simulink model "gm_final_heart_sym2_level3_hdl"  (R2021a)
settings: Solver=FixedStepDiscrete  StartTime=0.0  StopTime=10.0  RelTol=1e-3
libraries: hdlmdlgenlib x34
(part 1 of 3)
settings Model: Creator=Acer  LastModifiedBy=Acer
settings OptimizationCC: BlockReduction=off  ConditionallyExecuteInputs=off  DefaultParameterBehavior=Inlined
settings DebuggingCC: AlgebraicLoopMsg=error  InheritedTsInSrcMsg=none  SingleTaskRateTransMsg=error
settings HardwareCC: ProdBitPerPointer=32  ProdBitPerSizeT=32  ProdBitPerPtrDiffT=32  ProdLargestAtomicFloat=None  ProdIntDivRoundTo=Undefined  ProdEndianess=Unspecified  ProdWordSize=32  ProdHWDeviceType=ASIC/FPGA->ASIC/FPGA  TargetBitPerPointer=64  TargetBitPerSizeT=64  TargetBitPerPtrDiffT=64  TargetLongLongMode=on  TargetIntDivRoundTo=Zero  TargetEndianess=LittleEndian  TargetWordSize=64  TargetHWDeviceType=Custom Processor->MATLAB Host Computer  ProdEqTarget=off

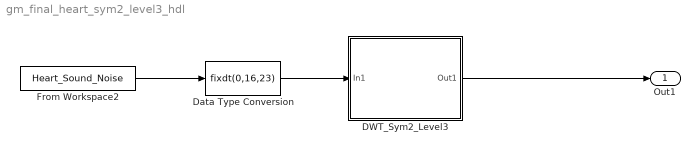
== system gm_final_heart_sym2_level3_hdl ==
  DWT_Sym2_Level3 : Subsystem
  Data Type Conversion : DataTypeConversion  OutDataTypeStr=fixdt(0,16,23)
  From Workspace2 : FromWorkspace  VariableName=Heart_Sound_Noise  OutDataTypeStr=double  SampleTime=1/44100
  Out1 : Outport  OutDataTypeStr=fixdt(1,16,22)
  wires:
  Data Type Conversion/1 -> DWT_Sym2_Level3/1(In1)
  DWT_Sym2_Level3/1(Out1) -> Out1/1
  From Workspace2/1 -> Data Type Conversion/1

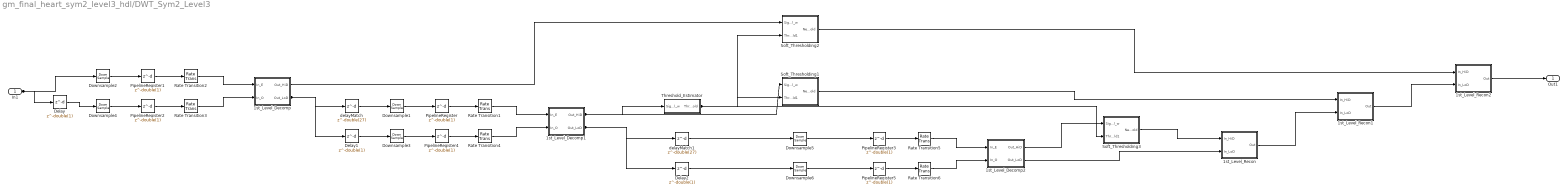
== system gm_final_heart_sym2_level3_hdl/DWT_Sym2_Level3 ==
  In1 : Inport  OutDataTypeStr=fixdt(0, 16, 23)  PortDimensions=1  SampleTime=2.26757369614512e-05
  1st_Level_Decomp : Subsystem
  1st_Level_Decomp1 : Subsystem
  1st_Level_Decomp2 : Subsystem
  1st_Level_Recon : Subsystem
  1st_Level_Recon1 : Subsystem
  1st_Level_Recon2 : Subsystem
  Delay : Delay  DelayLength=double(1)  InitialCondition=0  SampleTime=2.26757369614512e-05
  Delay1 : Delay  DelayLength=double(1)  InitialCondition=0  SampleTime=2.26757369614512e-05
  Delay2 : Delay  DelayLength=double(1)  InitialCondition=0  SampleTime=2.26757369614512e-05
  Downsample{1..2,4..5} (4 alike) : DownSample  N=double(30)  phase=double(0)  RateOptions=Allow multirate processing
  Downsample3 : DownSample  N=double(30)  phase=double(3)  RateOptions=Allow multirate processing
  Downsample6 : DownSample  N=double(30)  phase=double(3)  RateOptions=Allow multirate processing
  PipelineRegister{,1..5} (6 alike) : Delay  DelayLength=double(1)  InitialCondition=0  SampleTime=0.000680272108843537
  Rate Transition{1..6} (6 alike) : RateTransition  InitialCondition=double(0)  OutPortSampleTimeOpt=Multiple of input port sample time  OutPortSampleTimeMultiple=1/30
  Soft_Thresholding1 : Subsystem
  Soft_Thresholding2 : Subsystem
  Soft_Thresholding3 : Subsystem
  Threshold_Estimator : Subsystem
  delayMatch : Delay  DelayLength=double(27)  InitialCondition=0  SampleTime=2.26757369614512e-05
  delayMatch1 : Delay  DelayLength=double(27)  InitialCondition=0  SampleTime=2.26757369614512e-05
  Out1 : Outport  OutDataTypeStr=fixdt(1,16,22)  SampleTime=2.26757369614512e-05
  wires:
  In1/1 -> Downsample2/1, Delay/1
  1st_Level_Decomp/1(Out_HiD) -> Soft_Thresholding2/1(Signal_w)
  delayMatch/1 -> Downsample1/1
  1st_Level_Decomp1/1(Out_HiD) -> Soft_Thresholding1/1(Signal_w), Threshold_Estimator/1(Signal_w)
  delayMatch1/1 -> Downsample5/1
  1st_Level_Decomp2/1(Out_HiD) -> Soft_Thresholding3/1(Signal_w)
  1st_Level_Decomp2/2(Out_LoD) -> 1st_Level_Recon/2(In_LoD)
  1st_Level_Recon/1(Out) -> 1st_Level_Recon1/2(In_LoD)
  1st_Level_Recon1/1(Out) -> 1st_Level_Recon2/2(In_LoD)
  1st_Level_Recon2/1(Out) -> Out1/1
  Delay/1 -> Downsample4/1
  PipelineRegister/1 -> Rate Transition1/1
  PipelineRegister1/1 -> Rate Transition2/1
  PipelineRegister4/1 -> Rate Transition4/1
  PipelineRegister2/1 -> Rate Transition3/1
  PipelineRegister3/1 -> Rate Transition5/1
  PipelineRegister5/1 -> Rate Transition6/1
  Rate Transition1/1 -> 1st_Level_Decomp1/1(In_E)
  Rate Transition2/1 -> 1st_Level_Decomp/1(In_E)
  Rate Transition3/1 -> 1st_Level_Decomp/2(In_O)
  Rate Transition4/1 -> 1st_Level_Decomp1/2(In_O)
  Rate Transition5/1 -> 1st_Level_Decomp2/1(In_E)
  Rate Transition6/1 -> 1st_Level_Decomp2/2(In_O)
  Soft_Thresholding1/1(New_Threshold) -> 1st_Level_Recon1/1(In_HiD)
  Soft_Thresholding2/1(New_Threshold) -> 1st_Level_Recon2/1(In_HiD)
  Soft_Thresholding3/1(New_Threshold) -> 1st_Level_Recon/1(In_HiD)
  Threshold_Estimator/1(Threshold) -> Soft_Thresholding3/2(Threshold1), Soft_Thresholding2/2(Threshold1), Soft_Thresholding1/2(Threshold1)
  1st_Level_Decomp/2(Out_LoD) -> delayMatch/1, Delay1/1
  Delay1/1 -> Downsample3/1
  1st_Level_Decomp1/2(Out_LoD) -> delayMatch1/1, Delay2/1
  Delay2/1 -> Downsample6/1
  Downsample1/1 -> PipelineRegister/1
  Downsample2/1 -> PipelineRegister1/1
  Downsample4/1 -> PipelineRegister2/1
  Downsample5/1 -> PipelineRegister3/1
  Downsample3/1 -> PipelineRegister4/1
  Downsample6/1 -> PipelineRegister5/1

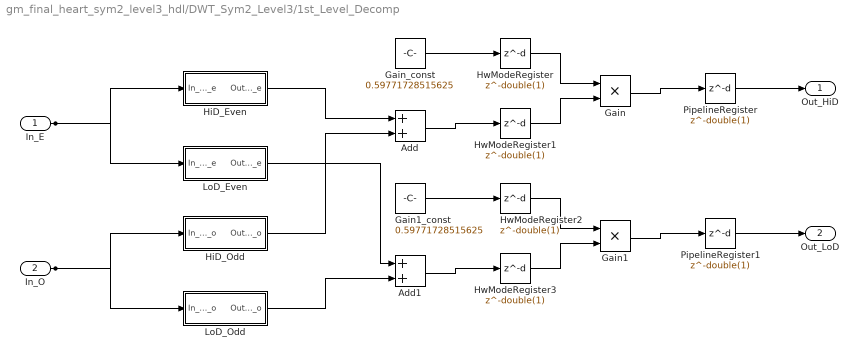
== system gm_final_heart_sym2_level3_hdl/DWT_Sym2_Level3/1st_Level_Decomp ==
  In_E : Inport  OutDataTypeStr=fixdt(0, 16, 23)  PortDimensions=1  SampleTime=2.26757369614512e-05
  In_O : Inport  Port=2  OutDataTypeStr=fixdt(0, 16, 23)  PortDimensions=1  SampleTime=2.26757369614512e-05
  Add : Sum  AccumDataTypeStr=fixdt(1, 16, 23)  OutDataTypeStr=fixdt(1, 16, 24)  SampleTime=2.26757369614512e-05
  Add1 : Sum  AccumDataTypeStr=fixdt(1, 16, 22)  OutDataTypeStr=fixdt(1, 16, 22)  SampleTime=2.26757369614512e-05
  Gain : Product  Inputs=**  OutDataTypeStr=fixdt(1, 16, 24)  SampleTime=2.26757369614512e-05
  Gain1 : Product  Inputs=**  OutDataTypeStr=fixdt(1, 16, 22)  SampleTime=2.26757369614512e-05
  Gain1_const : Constant  Value=0.59771728515625  OutDataTypeStr=fixdt(0, 16, 16)  SampleTime=2.26757369614512e-05
  Gain_const : Constant  Value=0.59771728515625  OutDataTypeStr=fixdt(0, 16, 16)  SampleTime=2.26757369614512e-05
  HiD_Even : Subsystem
  HiD_Odd : Subsystem
  HwModeRegister{,1..3} (4 alike) : Delay  DelayLength=double(1)  InitialCondition=0  SampleTime=2.26757369614512e-05
  LoD_Even : Subsystem
  LoD_Odd : Subsystem
  PipelineRegister : Delay  DelayLength=double(1)  InitialCondition=0  SampleTime=2.26757369614512e-05
  PipelineRegister1 : Delay  DelayLength=double(1)  InitialCondition=0  SampleTime=2.26757369614512e-05
  Out_HiD : Outport  OutDataTypeStr=fixdt(1,16,24)  SampleTime=2.26757369614512e-05
  Out_LoD : Outport  Port=2  OutDataTypeStr=fixdt(1,16,22)  SampleTime=2.26757369614512e-05
  wires:
  Add/1 -> HwModeRegister1/1
  Add1/1 -> HwModeRegister3/1
  PipelineRegister/1 -> Out_HiD/1
  PipelineRegister1/1 -> Out_LoD/1
  HiD_Even/1(Out_HiD_e) -> Add/1
  HiD_Odd/1(Out_HiD_o) -> Add/2
  LoD_Even/1(Out_LoD_e) -> Add1/1
  LoD_Odd/1(Out_LoD_o) -> Add1/2
  Gain_const/1 -> HwModeRegister/1
  Gain1_const/1 -> HwModeRegister2/1
  In_E/1 -> HiD_Even/1(In_HiD_e), LoD_Even/1(In_LoD_e)
  In_O/1 -> HiD_Odd/1(In_HiD_o), LoD_Odd/1(In_LoD_o)
  Gain/1 -> PipelineRegister/1
  HwModeRegister/1 -> Gain/1
  HwModeRegister1/1 -> Gain/2
  Gain1/1 -> PipelineRegister1/1
  HwModeRegister2/1 -> Gain1/1
  HwModeRegister3/1 -> Gain1/2

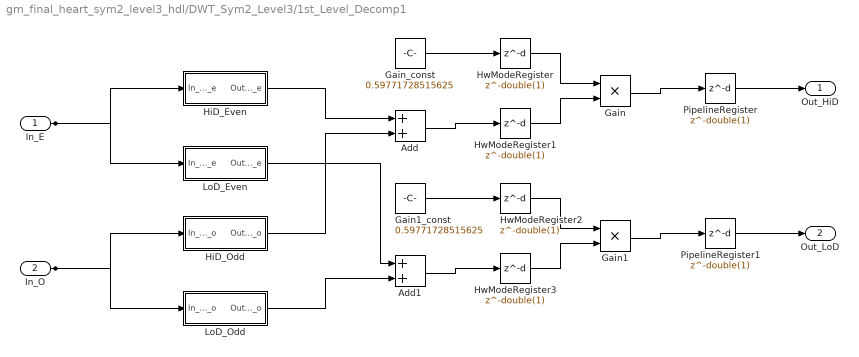
== system gm_final_heart_sym2_level3_hdl/DWT_Sym2_Level3/1st_Level_Decomp1 ==
  In_E : Inport  OutDataTypeStr=fixdt(1, 16, 22)  PortDimensions=1  SampleTime=2.26757369614512e-05
  In_O : Inport  Port=2  OutDataTypeStr=fixdt(1, 16, 22)  PortDimensions=1  SampleTime=2.26757369614512e-05
  Add : Sum  AccumDataTypeStr=fixdt(1, 16, 23)  OutDataTypeStr=fixdt(1, 16, 26)  SampleTime=2.26757369614512e-05
  Add1 : Sum  AccumDataTypeStr=fixdt(1, 16, 22)  OutDataTypeStr=fixdt(0, 16, 23)  SampleTime=2.26757369614512e-05
  Gain : Product  Inputs=**  OutDataTypeStr=fixdt(1, 16, 26)  SampleTime=2.26757369614512e-05
  Gain1 : Product  Inputs=**  OutDataTypeStr=fixdt(0, 16, 24)  SampleTime=2.26757369614512e-05
  Gain1_const : Constant  Value=0.59771728515625  OutDataTypeStr=fixdt(0, 16, 16)  SampleTime=2.26757369614512e-05
  Gain_const : Constant  Value=0.59771728515625  OutDataTypeStr=fixdt(0, 16, 16)  SampleTime=2.26757369614512e-05
  HiD_Even : Subsystem
  HiD_Odd : Subsystem
  HwModeRegister{,1..3} (4 alike) : Delay  DelayLength=double(1)  InitialCondition=0  SampleTime=2.26757369614512e-05
  LoD_Even : Subsystem
  LoD_Odd : Subsystem
  PipelineRegister : Delay  DelayLength=double(1)  InitialCondition=0  SampleTime=2.26757369614512e-05
  PipelineRegister1 : Delay  DelayLength=double(1)  InitialCondition=0  SampleTime=2.26757369614512e-05
  Out_HiD : Outport  OutDataTypeStr=fixdt(1,16,26)  SampleTime=2.26757369614512e-05
  Out_LoD : Outport  Port=2  OutDataTypeStr=fixdt(0,16,24)  SampleTime=2.26757369614512e-05
  wires:
  Add/1 -> HwModeRegister1/1
  Add1/1 -> HwModeRegister3/1
  PipelineRegister/1 -> Out_HiD/1
  PipelineRegister1/1 -> Out_LoD/1
  HiD_Even/1(Out_HiD_e) -> Add/1
  HiD_Odd/1(Out_HiD_o) -> Add/2
  LoD_Even/1(Out_LoD_e) -> Add1/1
  LoD_Odd/1(Out_LoD_o) -> Add1/2
  Gain_const/1 -> HwModeRegister/1
  Gain1_const/1 -> HwModeRegister2/1
  In_E/1 -> HiD_Even/1(In_HiD_e), LoD_Even/1(In_LoD_e)
  In_O/1 -> HiD_Odd/1(In_HiD_o), LoD_Odd/1(In_LoD_o)
  Gain/1 -> PipelineRegister/1
  HwModeRegister/1 -> Gain/1
  HwModeRegister1/1 -> Gain/2
  Gain1/1 -> PipelineRegister1/1
  HwModeRegister2/1 -> Gain1/1
  HwModeRegister3/1 -> Gain1/2

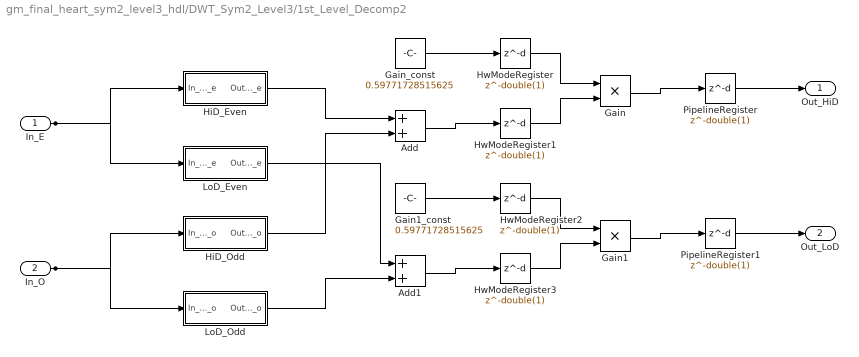
== system gm_final_heart_sym2_level3_hdl/DWT_Sym2_Level3/1st_Level_Decomp2 ==
  In_E : Inport  OutDataTypeStr=fixdt(0, 16, 24)  PortDimensions=1  SampleTime=2.26757369614512e-05
  In_O : Inport  Port=2  OutDataTypeStr=fixdt(0, 16, 24)  PortDimensions=1  SampleTime=2.26757369614512e-05
  Add : Sum  AccumDataTypeStr=fixdt(1, 16, 23)  OutDataTypeStr=fixdt(1, 16, 26)  SampleTime=2.26757369614512e-05
  Add1 : Sum  AccumDataTypeStr=fixdt(1, 16, 22)  OutDataTypeStr=fixdt(0, 16, 23)  SampleTime=2.26757369614512e-05
  Gain : Product  Inputs=**  OutDataTypeStr=fixdt(1, 16, 27)  SampleTime=2.26757369614512e-05
  Gain1 : Product  Inputs=**  OutDataTypeStr=fixdt(0, 16, 24)  SampleTime=2.26757369614512e-05
  Gain1_const : Constant  Value=0.59771728515625  OutDataTypeStr=fixdt(0, 16, 16)  SampleTime=2.26757369614512e-05
  Gain_const : Constant  Value=0.59771728515625  OutDataTypeStr=fixdt(0, 16, 16)  SampleTime=2.26757369614512e-05
  HiD_Even : Subsystem
  HiD_Odd : Subsystem
  HwModeRegister{,1..3} (4 alike) : Delay  DelayLength=double(1)  InitialCondition=0  SampleTime=2.26757369614512e-05
  LoD_Even : Subsystem
  LoD_Odd : Subsystem
  PipelineRegister : Delay  DelayLength=double(1)  InitialCondition=0  SampleTime=2.26757369614512e-05
  PipelineRegister1 : Delay  DelayLength=double(1)  InitialCondition=0  SampleTime=2.26757369614512e-05
  Out_HiD : Outport  OutDataTypeStr=fixdt(1,16,27)  SampleTime=2.26757369614512e-05
  Out_LoD : Outport  Port=2  OutDataTypeStr=fixdt(0,16,24)  SampleTime=2.26757369614512e-05
  wires:
  Add/1 -> HwModeRegister1/1
  Add1/1 -> HwModeRegister3/1
  PipelineRegister/1 -> Out_HiD/1
  PipelineRegister1/1 -> Out_LoD/1
  HiD_Even/1(Out_HiD_e) -> Add/1
  HiD_Odd/1(Out_HiD_o) -> Add/2
  LoD_Even/1(Out_LoD_e) -> Add1/1
  LoD_Odd/1(Out_LoD_o) -> Add1/2
  Gain_const/1 -> HwModeRegister/1
  Gain1_const/1 -> HwModeRegister2/1
  In_E/1 -> HiD_Even/1(In_HiD_e), LoD_Even/1(In_LoD_e)
  In_O/1 -> HiD_Odd/1(In_HiD_o), LoD_Odd/1(In_LoD_o)
  Gain/1 -> PipelineRegister/1
  HwModeRegister/1 -> Gain/1
  HwModeRegister1/1 -> Gain/2
  Gain1/1 -> PipelineRegister1/1
  HwModeRegister2/1 -> Gain1/1
  HwModeRegister3/1 -> Gain1/2

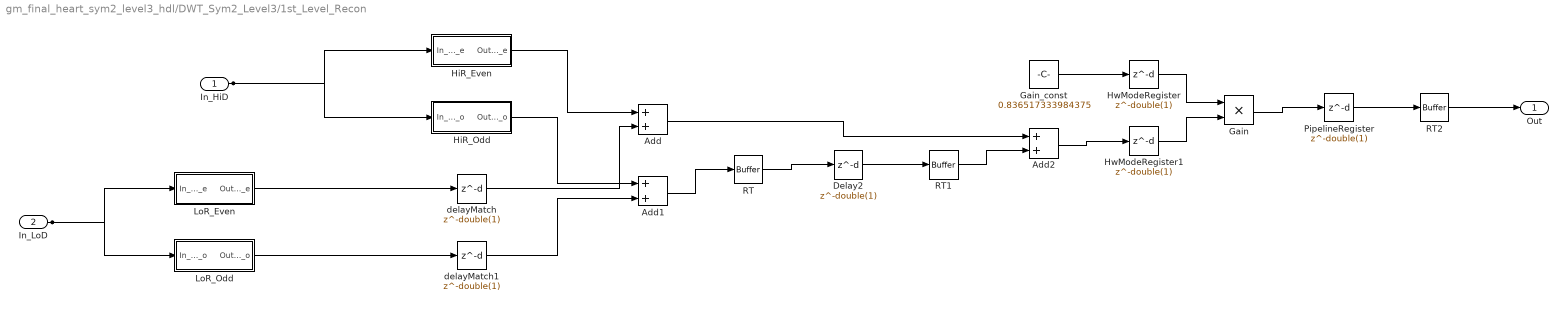
== system gm_final_heart_sym2_level3_hdl/DWT_Sym2_Level3/1st_Level_Recon ==
  In_HiD : Inport  OutDataTypeStr=fixdt(1, 16, 27)  PortDimensions=1  SampleTime=2.26757369614512e-05
  In_LoD : Inport  Port=2  OutDataTypeStr=fixdt(0, 16, 24)  PortDimensions=1  SampleTime=2.26757369614512e-05
  Add : Sum  AccumDataTypeStr=fixdt(1, 16, 23)  OutDataTypeStr=fixdt(1, 16, 23)  SampleTime=2.26757369614512e-05
  Add1 : Sum  AccumDataTypeStr=fixdt(1, 16, 23)  OutDataTypeStr=fixdt(1, 16, 23)  SampleTime=2.26757369614512e-05
  Add2 : Sum  AccumDataTypeStr=fixdt(1, 16, 22)  OutDataTypeStr=fixdt(1, 16, 22)  SampleTime=2.26757369614512e-05
  Delay2 : Delay  DelayLength=double(1)  InitialCondition=0  SampleTime=2.26757369614512e-05
  Gain : Product  Inputs=**  OutDataTypeStr=fixdt(1, 16, 23)  SampleTime=2.26757369614512e-05
  Gain_const : Constant  Value=0.836517333984375  OutDataTypeStr=fixdt(0, 16, 16)  SampleTime=2.26757369614512e-05
  HiR_Even : Subsystem
  HiR_Odd : Subsystem
  HwModeRegister : Delay  DelayLength=double(1)  InitialCondition=0  SampleTime=2.26757369614512e-05
  HwModeRegister1 : Delay  DelayLength=double(1)  InitialCondition=0  SampleTime=2.26757369614512e-05
  LoR_Even : Subsystem
  LoR_Odd : Subsystem
  PipelineRegister : Delay  DelayLength=double(1)  InitialCondition=0  SampleTime=2.26757369614512e-05
  RT : hdlmdlgenlib/Buffer
      settings: SourceProductBaseCode=SL
  RT1 : hdlmdlgenlib/Buffer
      settings: SourceProductBaseCode=SL
  RT2 : hdlmdlgenlib/Buffer
      settings: SourceProductBaseCode=SL
  delayMatch : Delay  DelayLength=double(1)  InitialCondition=0  SampleTime=2.26757369614512e-05
  delayMatch1 : Delay  DelayLength=double(1)  InitialCondition=0  SampleTime=2.26757369614512e-05
  Out : Outport  OutDataTypeStr=fixdt(1,16,23)  SampleTime=2.26757369614512e-05
  wires:
  Add/1 -> Add2/1
  Add1/1 -> RT/1
  Add2/1 -> HwModeRegister1/1
  Delay2/1 -> RT1/1
  PipelineRegister/1 -> RT2/1
  HiR_Even/1(Out_HiR_e) -> Add/1
  HiR_Odd/1(Out_HiR_o) -> Add1/1
  delayMatch/1 -> Add/2
  delayMatch1/1 -> Add1/2
  RT/1 -> Delay2/1
  RT1/1 -> Add2/2
  RT2/1 -> Out/1
  Gain_const/1 -> HwModeRegister/1
  In_HiD/1 -> HiR_Even/1(In_HiR_e), HiR_Odd/1(In_HiR_o)
  In_LoD/1 -> LoR_Odd/1(In_LoR_o), LoR_Even/1(In_LoR_e)
  LoR_Even/1(Out_LoR_e) -> delayMatch/1
  LoR_Odd/1(Out_HiR_o) -> delayMatch1/1
  Gain/1 -> PipelineRegister/1
  HwModeRegister/1 -> Gain/1
  HwModeRegister1/1 -> Gain/2

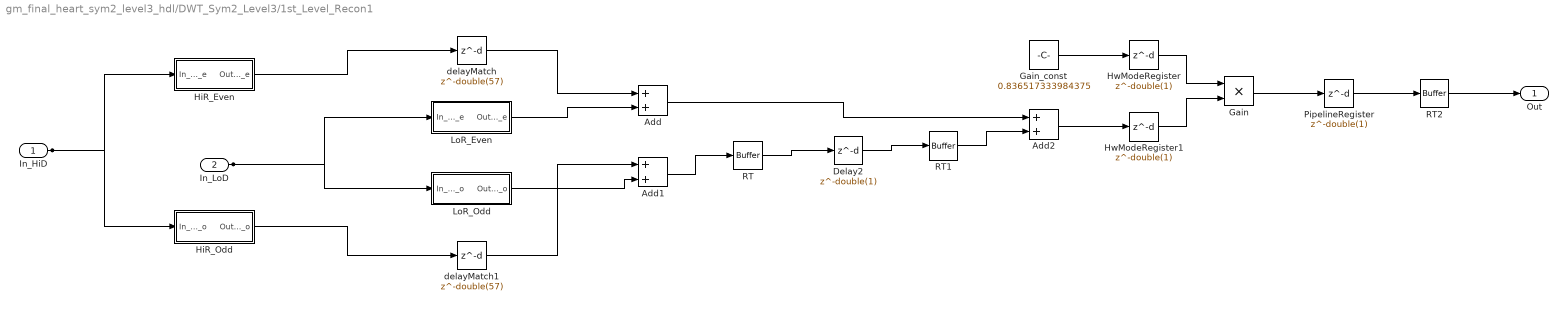
== system gm_final_heart_sym2_level3_hdl/DWT_Sym2_Level3/1st_Level_Recon1 ==
  In_HiD : Inport  OutDataTypeStr=fixdt(1, 16, 27)  PortDimensions=1  SampleTime=2.26757369614512e-05
  In_LoD : Inport  Port=2  OutDataTypeStr=fixdt(1, 16, 23)  PortDimensions=1  SampleTime=2.26757369614512e-05
  Add : Sum  AccumDataTypeStr=fixdt(1, 16, 23)  OutDataTypeStr=fixdt(1, 16, 23)  SampleTime=2.26757369614512e-05
  Add1 : Sum  AccumDataTypeStr=fixdt(1, 16, 23)  OutDataTypeStr=fixdt(1, 16, 23)  SampleTime=2.26757369614512e-05
  Add2 : Sum  AccumDataTypeStr=fixdt(1, 16, 22)  OutDataTypeStr=fixdt(1, 16, 22)  SampleTime=2.26757369614512e-05
  Delay2 : Delay  DelayLength=double(1)  InitialCondition=0  SampleTime=2.26757369614512e-05
  Gain : Product  Inputs=**  OutDataTypeStr=fixdt(1, 16, 22)  SampleTime=2.26757369614512e-05
  Gain_const : Constant  Value=0.836517333984375  OutDataTypeStr=fixdt(0, 16, 16)  SampleTime=2.26757369614512e-05
  HiR_Even : Subsystem
  HiR_Odd : Subsystem
  HwModeRegister : Delay  DelayLength=double(1)  InitialCondition=0  SampleTime=2.26757369614512e-05
  HwModeRegister1 : Delay  DelayLength=double(1)  InitialCondition=0  SampleTime=2.26757369614512e-05
  LoR_Even : Subsystem
  LoR_Odd : Subsystem
  PipelineRegister : Delay  DelayLength=double(1)  InitialCondition=0  SampleTime=2.26757369614512e-05
  RT : hdlmdlgenlib/Buffer
      settings: SourceProductBaseCode=SL
  RT1 : hdlmdlgenlib/Buffer
      settings: SourceProductBaseCode=SL
  RT2 : hdlmdlgenlib/Buffer
      settings: SourceProductBaseCode=SL
  delayMatch : Delay  DelayLength=double(57)  InitialCondition=0  SampleTime=2.26757369614512e-05
  delayMatch1 : Delay  DelayLength=double(57)  InitialCondition=0  SampleTime=2.26757369614512e-05
  Out : Outport  OutDataTypeStr=fixdt(1,16,22)  SampleTime=2.26757369614512e-05
  wires:
  Add/1 -> Add2/1
  Add1/1 -> RT/1
  Add2/1 -> HwModeRegister1/1
  Delay2/1 -> RT1/1
  PipelineRegister/1 -> RT2/1
  delayMatch/1 -> Add/1
  delayMatch1/1 -> Add1/1
  LoR_Even/1(Out_LoR_e) -> Add/2
  LoR_Odd/1(Out_HiR_o) -> Add1/2
  RT/1 -> Delay2/1
  RT1/1 -> Add2/2
  RT2/1 -> Out/1
  Gain_const/1 -> HwModeRegister/1
  In_HiD/1 -> HiR_Even/1(In_HiR_e), HiR_Odd/1(In_HiR_o)
  In_LoD/1 -> LoR_Odd/1(In_LoR_o), LoR_Even/1(In_LoR_e)
  HiR_Even/1(Out_HiR_e) -> delayMatch/1
  HiR_Odd/1(Out_HiR_o) -> delayMatch1/1
  Gain/1 -> PipelineRegister/1
  HwModeRegister/1 -> Gain/1
  HwModeRegister1/1 -> Gain/2

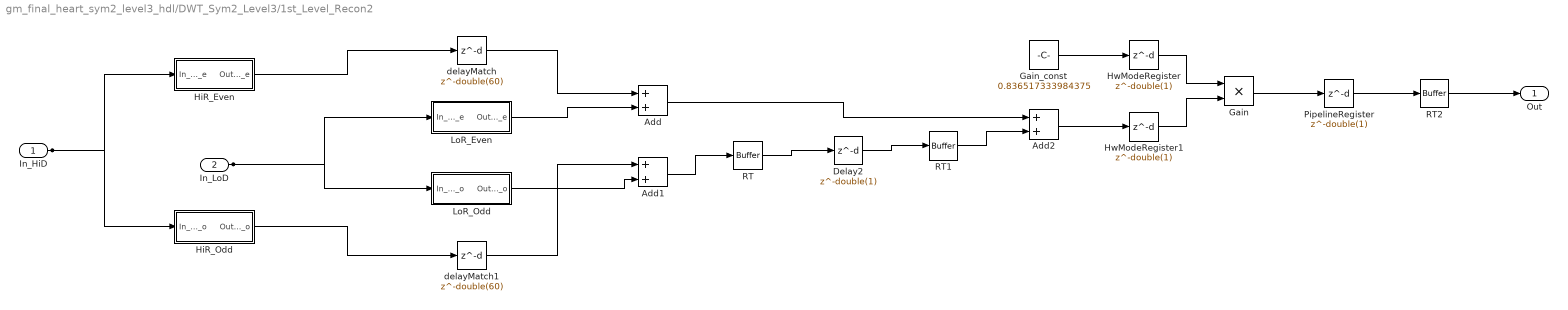
== system gm_final_heart_sym2_level3_hdl/DWT_Sym2_Level3/1st_Level_Recon2 ==
  In_HiD : Inport  OutDataTypeStr=fixdt(1, 16, 28)  PortDimensions=1  SampleTime=2.26757369614512e-05
  In_LoD : Inport  Port=2  OutDataTypeStr=fixdt(1, 16, 22)  PortDimensions=1  SampleTime=2.26757369614512e-05
  Add : Sum  AccumDataTypeStr=fixdt(1, 16, 23)  OutDataTypeStr=fixdt(1, 16, 23)  SampleTime=2.26757369614512e-05
  Add1 : Sum  AccumDataTypeStr=fixdt(1, 16, 23)  OutDataTypeStr=fixdt(1, 16, 23)  SampleTime=2.26757369614512e-05
  Add2 : Sum  AccumDataTypeStr=fixdt(1, 16, 22)  OutDataTypeStr=fixdt(1, 16, 22)  SampleTime=2.26757369614512e-05
  Delay2 : Delay  DelayLength=double(1)  InitialCondition=0  SampleTime=2.26757369614512e-05
  Gain : Product  Inputs=**  OutDataTypeStr=fixdt(1, 16, 22)  SampleTime=2.26757369614512e-05
  Gain_const : Constant  Value=0.836517333984375  OutDataTypeStr=fixdt(0, 16, 16)  SampleTime=2.26757369614512e-05
  HiR_Even : Subsystem
  HiR_Odd : Subsystem
  HwModeRegister : Delay  DelayLength=double(1)  InitialCondition=0  SampleTime=2.26757369614512e-05
  HwModeRegister1 : Delay  DelayLength=double(1)  InitialCondition=0  SampleTime=2.26757369614512e-05
  LoR_Even : Subsystem
  LoR_Odd : Subsystem
  PipelineRegister : Delay  DelayLength=double(1)  InitialCondition=0  SampleTime=2.26757369614512e-05
  RT : hdlmdlgenlib/Buffer
      settings: SourceProductBaseCode=SL
  RT1 : hdlmdlgenlib/Buffer
      settings: SourceProductBaseCode=SL
  RT2 : hdlmdlgenlib/Buffer
      settings: SourceProductBaseCode=SL
  delayMatch : Delay  DelayLength=double(60)  InitialCondition=0  SampleTime=2.26757369614512e-05
  delayMatch1 : Delay  DelayLength=double(60)  InitialCondition=0  SampleTime=2.26757369614512e-05
  Out : Outport  OutDataTypeStr=fixdt(1,16,22)  SampleTime=2.26757369614512e-05
  wires:
  Add/1 -> Add2/1
  Add1/1 -> RT/1
  Add2/1 -> HwModeRegister1/1
  Delay2/1 -> RT1/1
  PipelineRegister/1 -> RT2/1
  delayMatch/1 -> Add/1
  delayMatch1/1 -> Add1/1
  LoR_Even/1(Out_LoR_e) -> Add/2
  LoR_Odd/1(Out_HiR_o) -> Add1/2
  RT/1 -> Delay2/1
  RT1/1 -> Add2/2
  RT2/1 -> Out/1
  Gain_const/1 -> HwModeRegister/1
  In_HiD/1 -> HiR_Even/1(In_HiR_e), HiR_Odd/1(In_HiR_o)
  In_LoD/1 -> LoR_Odd/1(In_LoR_o), LoR_Even/1(In_LoR_e)
  HiR_Even/1(Out_HiR_e) -> delayMatch/1
  HiR_Odd/1(Out_HiR_o) -> delayMatch1/1
  Gain/1 -> PipelineRegister/1
  HwModeRegister/1 -> Gain/1
  HwModeRegister1/1 -> Gain/2

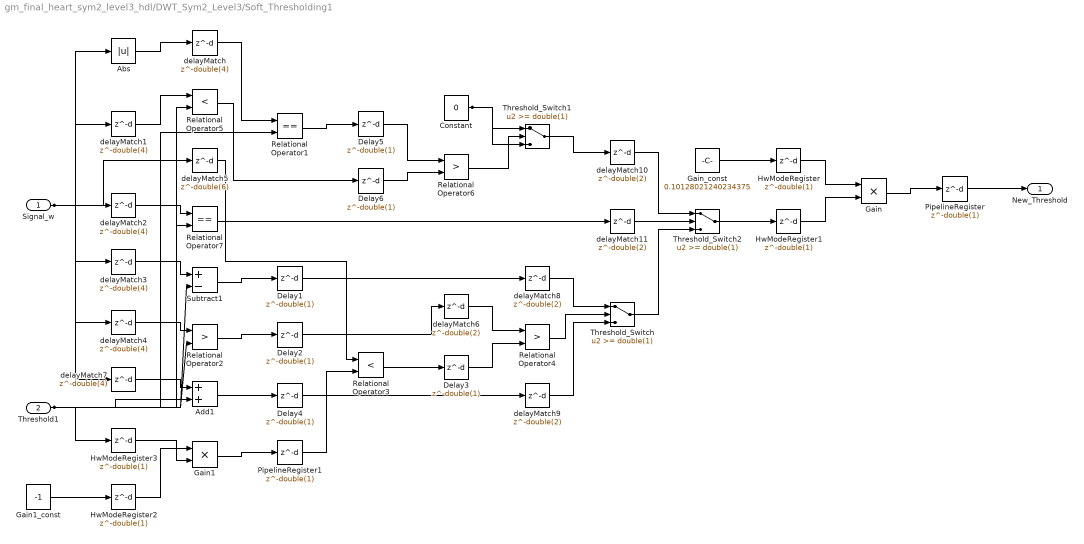
== system gm_final_heart_sym2_level3_hdl/DWT_Sym2_Level3/Soft_Thresholding1 ==
  Signal_w : Inport  OutDataTypeStr=fixdt(1, 16, 26)  PortDimensions=1  SampleTime=2.26757369614512e-05
  Threshold1 : Inport  Port=2  OutDataTypeStr=fixdt(0, 16, 25)  PortDimensions=1  SampleTime=2.26757369614512e-05
  Abs : Abs  SampleTime=2.26757369614512e-05  OutDataTypeStr=fixdt(0, 16, 27)
  Add1 : Sum  AccumDataTypeStr=fixdt(1, 16, 24)  OutDataTypeStr=fixdt(1, 16, 24)  SampleTime=2.26757369614512e-05
  Constant : Constant  Value=0  OutDataTypeStr=fixdt(1, 16, 4)  SampleTime=2.26757369614512e-05
  Delay{1..6} (6 alike) : Delay  DelayLength=double(1)  InitialCondition=0  SampleTime=2.26757369614512e-05
  Gain : Product  Inputs=**  OutDataTypeStr=fixdt(1, 16, 27)  SampleTime=2.26757369614512e-05
  Gain1 : Product  Inputs=**  OutDataTypeStr=fixdt(1, 16, 15)  SampleTime=2.26757369614512e-05
  Gain1_const : Constant  Value=-1  OutDataTypeStr=fixdt(1, 16, 15)  SampleTime=2.26757369614512e-05
  Gain_const : Constant  Value=0.10128021240234375  OutDataTypeStr=fixdt(0, 16, 19)  SampleTime=2.26757369614512e-05
  HwModeRegister{,1..3} (4 alike) : Delay  DelayLength=double(1)  InitialCondition=0  SampleTime=2.26757369614512e-05
  PipelineRegister : Delay  DelayLength=double(1)  InitialCondition=0  SampleTime=2.26757369614512e-05
  PipelineRegister1 : Delay  DelayLength=double(1)  InitialCondition=0  SampleTime=2.26757369614512e-05
  Relational Operator1 : RelationalOperator  Operator===  OutDataTypeStr=boolean  SampleTime=2.26757369614512e-05  RndMeth=Nearest
  Relational Operator2 : RelationalOperator  Operator=>  OutDataTypeStr=boolean  SampleTime=2.26757369614512e-05  RndMeth=Nearest
  Relational Operator3 : RelationalOperator  Operator=<  OutDataTypeStr=boolean  SampleTime=2.26757369614512e-05  RndMeth=Nearest
  Relational Operator4 : RelationalOperator  Operator=>  OutDataTypeStr=boolean  SampleTime=2.26757369614512e-05  RndMeth=Nearest
  Relational Operator5 : RelationalOperator  Operator=<  OutDataTypeStr=boolean  SampleTime=2.26757369614512e-05  RndMeth=Nearest
  Relational Operator6 : RelationalOperator  Operator=>  OutDataTypeStr=boolean  SampleTime=2.26757369614512e-05  RndMeth=Nearest
  Relational Operator7 : RelationalOperator  Operator===  OutDataTypeStr=boolean  SampleTime=2.26757369614512e-05  RndMeth=Nearest
  Subtract1 : Sum  Inputs=+-  AccumDataTypeStr=fixdt(1, 16, 24)  OutDataTypeStr=fixdt(1, 16, 24)  SampleTime=2.26757369614512e-05
  Threshold_Switch : Switch  Threshold=double(1)  OutDataTypeStr=fixdt(1, 16, 24)  SampleTime=2.26757369614512e-05
  Threshold_Switch1 : Switch  Threshold=double(1)  OutDataTypeStr=fixdt(1, 16, 4)  SampleTime=2.26757369614512e-05
  Threshold_Switch2 : Switch  Threshold=double(1)  OutDataTypeStr=fixdt(1, 16, 24)  SampleTime=2.26757369614512e-05
  delayMatch{,1..4,7} (6 alike) : Delay  DelayLength=double(4)  InitialCondition=0  SampleTime=2.26757369614512e-05
  delayMatch{6,8..11} (5 alike) : Delay  DelayLength=double(2)  InitialCondition=0  SampleTime=2.26757369614512e-05
  delayMatch5 : Delay  DelayLength=double(6)  InitialCondition=0  SampleTime=2.26757369614512e-05
  New_Threshold : Outport  OutDataTypeStr=fixdt(1,16,27)  SampleTime=2.26757369614512e-05
  wires:
  delayMatch1/1 -> Relational Operator5/1
  delayMatch/1 -> Relational Operator1/1
  Add1/1 -> Delay4/1
  Constant/1 -> Threshold_Switch1/3, Threshold_Switch1/1
  delayMatch8/1 -> Threshold_Switch/1
  delayMatch6/1 -> Relational Operator4/1
  Delay3/1 -> Relational Operator4/2
  delayMatch9/1 -> Threshold_Switch/3
  Delay5/1 -> Relational Operator6/1
  Delay6/1 -> Relational Operator6/2
  PipelineRegister/1 -> New_Threshold/1
  PipelineRegister1/1 -> Relational Operator3/2
  Relational Operator1/1 -> Delay5/1
  Relational Operator2/1 -> Delay2/1
  Relational Operator3/1 -> Delay3/1
  Relational Operator4/1 -> Threshold_Switch/2
  Relational Operator5/1 -> Delay6/1
  Relational Operator6/1 -> Threshold_Switch1/2
  delayMatch11/1 -> Threshold_Switch2/2
  Subtract1/1 -> Delay1/1
  Threshold_Switch/1 -> Threshold_Switch2/3
  delayMatch10/1 -> Threshold_Switch2/1
  Threshold_Switch2/1 -> HwModeRegister1/1
  Gain_const/1 -> HwModeRegister/1
  Gain1_const/1 -> HwModeRegister2/1
  Signal_w/1 -> delayMatch7/1, delayMatch5/1, delayMatch4/1, delayMatch3/1, delayMatch2/1, delayMatch1/1, Abs/1
  Threshold1/1 -> Subtract1/2, Relational Operator7/2, Relational Operator5/2, Relational Operator2/2, Relational Operator1/2, Add1/2, HwModeRegister3/1
  Abs/1 -> delayMatch/1
  delayMatch2/1 -> Relational Operator7/1
  delayMatch3/1 -> Subtract1/1
  delayMatch4/1 -> Relational Operator2/1
  delayMatch5/1 -> Relational Operator3/1
  delayMatch7/1 -> Add1/1
  Delay2/1 -> delayMatch6/1
  Delay1/1 -> delayMatch8/1
  Delay4/1 -> delayMatch9/1
  Threshold_Switch1/1 -> delayMatch10/1
  Relational Operator7/1 -> delayMatch11/1
  Gain/1 -> PipelineRegister/1
  HwModeRegister/1 -> Gain/1
  HwModeRegister1/1 -> Gain/2
  Gain1/1 -> PipelineRegister1/1
  HwModeRegister2/1 -> Gain1/1
  HwModeRegister3/1 -> Gain1/2

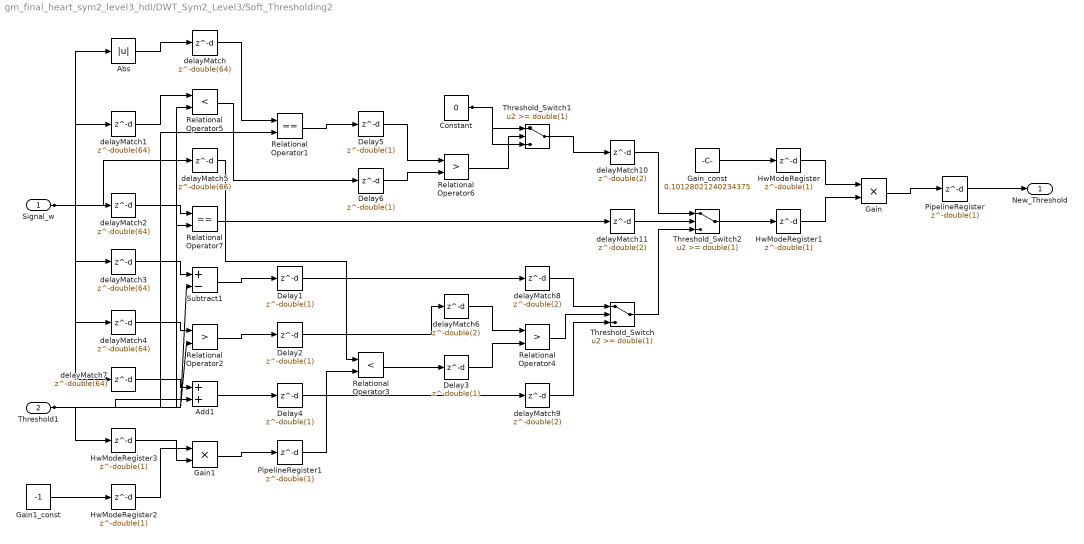
== system gm_final_heart_sym2_level3_hdl/DWT_Sym2_Level3/Soft_Thresholding2 ==
  Signal_w : Inport  OutDataTypeStr=fixdt(1, 16, 24)  PortDimensions=1  SampleTime=2.26757369614512e-05
  Threshold1 : Inport  Port=2  OutDataTypeStr=fixdt(0, 16, 25)  PortDimensions=1  SampleTime=2.26757369614512e-05
  Abs : Abs  SampleTime=2.26757369614512e-05  OutDataTypeStr=fixdt(0, 16, 25)
  Add1 : Sum  AccumDataTypeStr=fixdt(1, 16, 24)  OutDataTypeStr=fixdt(1, 16, 24)  SampleTime=2.26757369614512e-05
  Constant : Constant  Value=0  OutDataTypeStr=fixdt(1, 16, 4)  SampleTime=2.26757369614512e-05
  Delay{1..6} (6 alike) : Delay  DelayLength=double(1)  InitialCondition=0  SampleTime=2.26757369614512e-05
  Gain : Product  Inputs=**  OutDataTypeStr=fixdt(1, 16, 28)  SampleTime=2.26757369614512e-05
  Gain1 : Product  Inputs=**  OutDataTypeStr=fixdt(1, 16, 15)  SampleTime=2.26757369614512e-05
  Gain1_const : Constant  Value=-1  OutDataTypeStr=fixdt(1, 16, 15)  SampleTime=2.26757369614512e-05
  Gain_const : Constant  Value=0.10128021240234375  OutDataTypeStr=fixdt(0, 16, 19)  SampleTime=2.26757369614512e-05
  HwModeRegister{,1..3} (4 alike) : Delay  DelayLength=double(1)  InitialCondition=0  SampleTime=2.26757369614512e-05
  PipelineRegister : Delay  DelayLength=double(1)  InitialCondition=0  SampleTime=2.26757369614512e-05
  PipelineRegister1 : Delay  DelayLength=double(1)  InitialCondition=0  SampleTime=2.26757369614512e-05
  Relational Operator1 : RelationalOperator  Operator===  OutDataTypeStr=boolean  SampleTime=2.26757369614512e-05  RndMeth=Nearest
  Relational Operator2 : RelationalOperator  Operator=>  OutDataTypeStr=boolean  SampleTime=2.26757369614512e-05  RndMeth=Nearest
  Relational Operator3 : RelationalOperator  Operator=<  OutDataTypeStr=boolean  SampleTime=2.26757369614512e-05  RndMeth=Nearest
  Relational Operator4 : RelationalOperator  Operator=>  OutDataTypeStr=boolean  SampleTime=2.26757369614512e-05  RndMeth=Nearest
  Relational Operator5 : RelationalOperator  Operator=<  OutDataTypeStr=boolean  SampleTime=2.26757369614512e-05  RndMeth=Nearest
  Relational Operator6 : RelationalOperator  Operator=>  OutDataTypeStr=boolean  SampleTime=2.26757369614512e-05  RndMeth=Nearest
  Relational Operator7 : RelationalOperator  Operator===  OutDataTypeStr=boolean  SampleTime=2.26757369614512e-05  RndMeth=Nearest
  Subtract1 : Sum  Inputs=+-  AccumDataTypeStr=fixdt(1, 16, 24)  OutDataTypeStr=fixdt(1, 16, 24)  SampleTime=2.26757369614512e-05
  Threshold_Switch : Switch  Threshold=double(1)  OutDataTypeStr=fixdt(1, 16, 24)  SampleTime=2.26757369614512e-05
  Threshold_Switch1 : Switch  Threshold=double(1)  OutDataTypeStr=fixdt(1, 16, 4)  SampleTime=2.26757369614512e-05
  Threshold_Switch2 : Switch  Threshold=double(1)  OutDataTypeStr=fixdt(1, 16, 24)  SampleTime=2.26757369614512e-05
  delayMatch{,1..4,7} (6 alike) : Delay  DelayLength=double(64)  InitialCondition=0  SampleTime=2.26757369614512e-05
  delayMatch{6,8..11} (5 alike) : Delay  DelayLength=double(2)  InitialCondition=0  SampleTime=2.26757369614512e-05
  delayMatch5 : Delay  DelayLength=double(66)  InitialCondition=0  SampleTime=2.26757369614512e-05
  New_Threshold : Outport  OutDataTypeStr=fixdt(1,16,28)  SampleTime=2.26757369614512e-05
  wires:
  delayMatch1/1 -> Relational Operator5/1
  delayMatch/1 -> Relational Operator1/1
  Add1/1 -> Delay4/1
  Constant/1 -> Threshold_Switch1/3, Threshold_Switch1/1
  delayMatch8/1 -> Threshold_Switch/1
  delayMatch6/1 -> Relational Operator4/1
  Delay3/1 -> Relational Operator4/2
  delayMatch9/1 -> Threshold_Switch/3
  Delay5/1 -> Relational Operator6/1
  Delay6/1 -> Relational Operator6/2
  PipelineRegister/1 -> New_Threshold/1
  PipelineRegister1/1 -> Relational Operator3/2
  Relational Operator1/1 -> Delay5/1
  Relational Operator2/1 -> Delay2/1
  Relational Operator3/1 -> Delay3/1
  Relational Operator4/1 -> Threshold_Switch/2
  Relational Operator5/1 -> Delay6/1
  Relational Operator6/1 -> Threshold_Switch1/2
  delayMatch11/1 -> Threshold_Switch2/2
  Subtract1/1 -> Delay1/1
  Threshold_Switch/1 -> Threshold_Switch2/3
  delayMatch10/1 -> Threshold_Switch2/1
  Threshold_Switch2/1 -> HwModeRegister1/1
  Gain_const/1 -> HwModeRegister/1
  Gain1_const/1 -> HwModeRegister2/1
  Signal_w/1 -> delayMatch7/1, delayMatch5/1, delayMatch4/1, delayMatch3/1, delayMatch2/1, delayMatch1/1, Abs/1
  Threshold1/1 -> Subtract1/2, Relational Operator7/2, Relational Operator5/2, Relational Operator2/2, Relational Operator1/2, Add1/2, HwModeRegister3/1
  Abs/1 -> delayMatch/1
  delayMatch2/1 -> Relational Operator7/1
  delayMatch3/1 -> Subtract1/1
  delayMatch4/1 -> Relational Operator2/1
  delayMatch5/1 -> Relational Operator3/1
  delayMatch7/1 -> Add1/1
  Delay2/1 -> delayMatch6/1
  Delay1/1 -> delayMatch8/1
  Delay4/1 -> delayMatch9/1
  Threshold_Switch1/1 -> delayMatch10/1
  Relational Operator7/1 -> delayMatch11/1
  Gain/1 -> PipelineRegister/1
  HwModeRegister/1 -> Gain/1
  HwModeRegister1/1 -> Gain/2
  Gain1/1 -> PipelineRegister1/1
  HwModeRegister2/1 -> Gain1/1
  HwModeRegister3/1 -> Gain1/2

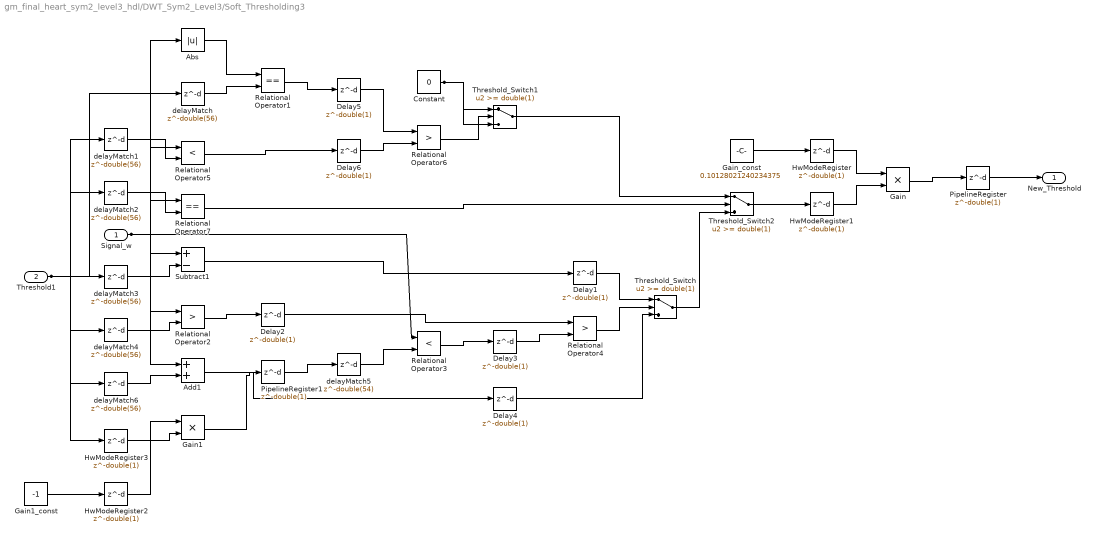
== system gm_final_heart_sym2_level3_hdl/DWT_Sym2_Level3/Soft_Thresholding3 ==
  Signal_w : Inport  OutDataTypeStr=fixdt(1, 16, 27)  PortDimensions=1  SampleTime=2.26757369614512e-05
  Threshold1 : Inport  Port=2  OutDataTypeStr=fixdt(0, 16, 25)  PortDimensions=1  SampleTime=2.26757369614512e-05
  Abs : Abs  SampleTime=2.26757369614512e-05  OutDataTypeStr=fixdt(0, 16, 28)
  Add1 : Sum  AccumDataTypeStr=fixdt(1, 16, 24)  OutDataTypeStr=fixdt(1, 16, 24)  SampleTime=2.26757369614512e-05
  Constant : Constant  Value=0  OutDataTypeStr=fixdt(1, 16, 4)  SampleTime=2.26757369614512e-05
  Delay{1..6} (6 alike) : Delay  DelayLength=double(1)  InitialCondition=0  SampleTime=2.26757369614512e-05
  Gain : Product  Inputs=**  OutDataTypeStr=fixdt(1, 16, 27)  SampleTime=2.26757369614512e-05
  Gain1 : Product  Inputs=**  OutDataTypeStr=fixdt(1, 16, 15)  SampleTime=2.26757369614512e-05
  Gain1_const : Constant  Value=-1  OutDataTypeStr=fixdt(1, 16, 15)  SampleTime=2.26757369614512e-05
  Gain_const : Constant  Value=0.10128021240234375  OutDataTypeStr=fixdt(0, 16, 19)  SampleTime=2.26757369614512e-05
  HwModeRegister{,1..3} (4 alike) : Delay  DelayLength=double(1)  InitialCondition=0  SampleTime=2.26757369614512e-05
  PipelineRegister : Delay  DelayLength=double(1)  InitialCondition=0  SampleTime=2.26757369614512e-05
  PipelineRegister1 : Delay  DelayLength=double(1)  InitialCondition=0  SampleTime=2.26757369614512e-05
  Relational Operator1 : RelationalOperator  Operator===  OutDataTypeStr=boolean  SampleTime=2.26757369614512e-05  RndMeth=Nearest
  Relational Operator2 : RelationalOperator  Operator=>  OutDataTypeStr=boolean  SampleTime=2.26757369614512e-05  RndMeth=Nearest
  Relational Operator3 : RelationalOperator  Operator=<  OutDataTypeStr=boolean  SampleTime=2.26757369614512e-05  RndMeth=Nearest
  Relational Operator4 : RelationalOperator  Operator=>  OutDataTypeStr=boolean  SampleTime=2.26757369614512e-05  RndMeth=Nearest
  Relational Operator5 : RelationalOperator  Operator=<  OutDataTypeStr=boolean  SampleTime=2.26757369614512e-05  RndMeth=Nearest
  Relational Operator6 : RelationalOperator  Operator=>  OutDataTypeStr=boolean  SampleTime=2.26757369614512e-05  RndMeth=Nearest
  Relational Operator7 : RelationalOperator  Operator===  OutDataTypeStr=boolean  SampleTime=2.26757369614512e-05  RndMeth=Nearest
  Subtract1 : Sum  Inputs=+-  AccumDataTypeStr=fixdt(1, 16, 24)  OutDataTypeStr=fixdt(1, 16, 24)  SampleTime=2.26757369614512e-05
  Threshold_Switch : Switch  Threshold=double(1)  OutDataTypeStr=fixdt(1, 16, 24)  SampleTime=2.26757369614512e-05
  Threshold_Switch1 : Switch  Threshold=double(1)  OutDataTypeStr=fixdt(1, 16, 4)  SampleTime=2.26757369614512e-05
  Threshold_Switch2 : Switch  Threshold=double(1)  OutDataTypeStr=fixdt(1, 16, 24)  SampleTime=2.26757369614512e-05
  delayMatch{,1..4,6} (6 alike) : Delay  DelayLength=double(56)  InitialCondition=0  SampleTime=2.26757369614512e-05
  delayMatch5 : Delay  DelayLength=double(54)  InitialCondition=0  SampleTime=2.26757369614512e-05
  New_Threshold : Outport  OutDataTypeStr=fixdt(1,16,27)  SampleTime=2.26757369614512e-05
  wires:
  delayMatch/1 -> Relational Operator1/2
  Abs/1 -> Relational Operator1/1
  Add1/1 -> Delay4/1
  Constant/1 -> Threshold_Switch1/3, Threshold_Switch1/1
  Delay1/1 -> Threshold_Switch/1
  Delay2/1 -> Relational Operator4/1
  Delay3/1 -> Relational Operator4/2
  Delay4/1 -> Threshold_Switch/3
  Delay5/1 -> Relational Operator6/1
  Delay6/1 -> Relational Operator6/2
  PipelineRegister/1 -> New_Threshold/1
  delayMatch5/1 -> Relational Operator3/2
  Relational Operator1/1 -> Delay5/1
  Relational Operator2/1 -> Delay2/1
  Relational Operator3/1 -> Delay3/1
  Relational Operator4/1 -> Threshold_Switch/2
  Relational Operator5/1 -> Delay6/1
  Relational Operator6/1 -> Threshold_Switch1/2
  Relational Operator7/1 -> Threshold_Switch2/2
  Subtract1/1 -> Delay1/1
  Threshold_Switch/1 -> Threshold_Switch2/3
  Threshold_Switch1/1 -> Threshold_Switch2/1
  Threshold_Switch2/1 -> HwModeRegister1/1
  Gain_const/1 -> HwModeRegister/1
  Gain1_const/1 -> HwModeRegister2/1
  Signal_w/1 -> Subtract1/1, Relational Operator7/1, Relational Operator5/1, Relational Operator3/1, Relational Operator2/1, Add1/1, Abs/1
  Threshold1/1 -> delayMatch6/1, delayMatch4/1, delayMatch3/1, delayMatch2/1, delayMatch1/1, delayMatch/1, HwModeRegister3/1
  delayMatch1/1 -> Relational Operator5/2
  delayMatch2/1 -> Relational Operator7/2
  delayMatch3/1 -> Subtract1/2
  delayMatch4/1 -> Relational Operator2/2
  delayMatch6/1 -> Add1/2
  PipelineRegister1/1 -> delayMatch5/1
  Gain/1 -> PipelineRegister/1
  HwModeRegister/1 -> Gain/1
  HwModeRegister1/1 -> Gain/2
  Gain1/1 -> PipelineRegister1/1
  HwModeRegister2/1 -> Gain1/1
  HwModeRegister3/1 -> Gain1/2

== system gm_final_heart_sym2_level3_hdl/DWT_Sym2_Level3/Threshold_Estimator ==
  Signal_w : Inport  OutDataTypeStr=fixdt(1, 16, 26)  PortDimensions=1  SampleTime=2.26757369614512e-05
  Absolute_Value1 : Subsystem
  HwModeRegister : Delay  DelayLength=double(1)  InitialCondition=0  SampleTime=2.26757369614512e-05
  HwModeRegister1 : Delay  DelayLength=double(1)  InitialCondition=0  SampleTime=2.26757369614512e-05
  Length : Constant  Value=4.936767578125  OutDataTypeStr=fixdt(0, 16, 13)  SampleTime=2.26757369614512e-05
  Median2 : Subsystem
  Multiply : Product  Inputs=**  OutDataTypeStr=fixdt(0, 16, 25)  SampleTime=2.26757369614512e-05
  PipelineRegister : Delay  DelayLength=double(1)  InitialCondition=0  SampleTime=2.26757369614512e-05
  Threshold : Outport  OutDataTypeStr=fixdt(0,16,25)  SampleTime=2.26757369614512e-05  VectorParamsAs1DForOutWhenUnconnected=off
  wires:
  Absolute_Value1/1(Out_Abs) -> Median2/1(Signal_w3)
  Length/1 -> HwModeRegister1/1
  Median2/1(Median) -> HwModeRegister/1
  PipelineRegister/1 -> Threshold/1
  Signal_w/1 -> Absolute_Value1/1(Signal_w4)
  Multiply/1 -> PipelineRegister/1
  HwModeRegister/1 -> Multiply/1
  HwModeRegister1/1 -> Multiply/2

== system gm_final_heart_sym2_level3_hdl/DWT_Sym2_Level3/1st_Level_Decomp/HiD_Even ==
  In_HiD_e : Inport  OutDataTypeStr=fixdt(0, 16, 23)  PortDimensions=1  SampleTime=2.26757369614512e-05
  Add : Sum  AccumDataTypeStr=fixdt(1, 16, 15)  OutDataTypeStr=fixdt(1, 16, 15)  SampleTime=2.26757369614512e-05
  Delay : Delay  DelayLength=double(1)  InitialCondition=0  SampleTime=2.26757369614512e-05
  HiD_0 : Constant  Value=-0.4829559326171875  OutDataTypeStr=fixdt(1, 16, 16)  SampleTime=2.26757369614512e-05
  HiD_2 : Constant  Value=-0.22414398193359375  OutDataTypeStr=fixdt(1, 16, 17)  SampleTime=2.26757369614512e-05
  HwModeRegister{,1..3} (4 alike) : Delay  DelayLength=double(1)  InitialCondition=0  SampleTime=2.26757369614512e-05
  Multiply : Product  Inputs=**  OutDataTypeStr=fixdt(1, 16, 15)  SampleTime=2.26757369614512e-05
  Multiply1 : Product  Inputs=**  OutDataTypeStr=fixdt(1, 16, 15)  SampleTime=2.26757369614512e-05
  PipelineRegister : Delay  DelayLength=double(1)  InitialCondition=0  SampleTime=2.26757369614512e-05
  PipelineRegister1 : Delay  DelayLength=double(1)  InitialCondition=0  SampleTime=2.26757369614512e-05
  Rate Transition : hdlmdlgenlib/Buffer
      settings: SourceProductBaseCode=SL
  delayMatch : Delay  DelayLength=double(1)  InitialCondition=0  SampleTime=2.26757369614512e-05
  Out_HiD_e : Outport  OutDataTypeStr=fixdt(1,16,15)  SampleTime=2.26757369614512e-05  VectorParamsAs1DForOutWhenUnconnected=off
  wires:
  Add/1 -> Out_HiD_e/1
  Delay/1 -> Rate Transition/1
  HiD_0/1 -> HwModeRegister/1
  HiD_2/1 -> HwModeRegister2/1
  PipelineRegister/1 -> Add/1
  delayMatch/1 -> Add/2
  Rate Transition/1 -> HwModeRegister3/1
  In_HiD_e/1 -> Delay/1, HwModeRegister1/1
  PipelineRegister1/1 -> delayMatch/1
  Multiply/1 -> PipelineRegister/1
  HwModeRegister/1 -> Multiply/1
  HwModeRegister1/1 -> Multiply/2
  Multiply1/1 -> PipelineRegister1/1
  HwModeRegister2/1 -> Multiply1/1
  HwModeRegister3/1 -> Multiply1/2

== system gm_final_heart_sym2_level3_hdl/DWT_Sym2_Level3/1st_Level_Decomp/HiD_Odd ==
  In_HiD_o : Inport  OutDataTypeStr=fixdt(0, 16, 23)  PortDimensions=1  SampleTime=2.26757369614512e-05
  Add : Sum  AccumDataTypeStr=fixdt(1, 16, 22)  OutDataTypeStr=fixdt(1, 16, 23)  SampleTime=2.26757369614512e-05
  Delay : Delay  DelayLength=double(1)  InitialCondition=0  SampleTime=2.26757369614512e-05
  HiD_1 : Constant  Value=0.836517333984375  OutDataTypeStr=fixdt(0, 16, 16)  SampleTime=2.26757369614512e-05
  HiD_3 : Constant  Value=-0.1294097900390625  OutDataTypeStr=fixdt(1, 16, 17)  SampleTime=2.26757369614512e-05
  HwModeRegister{,1..3} (4 alike) : Delay  DelayLength=double(1)  InitialCondition=0  SampleTime=2.26757369614512e-05
  Multiply : Product  Inputs=**  OutDataTypeStr=fixdt(0, 16, 23)  SampleTime=2.26757369614512e-05
  Multiply1 : Product  Inputs=**  OutDataTypeStr=fixdt(1, 16, 15)  SampleTime=2.26757369614512e-05
  PipelineRegister : Delay  DelayLength=double(1)  InitialCondition=0  SampleTime=2.26757369614512e-05
  PipelineRegister1 : Delay  DelayLength=double(1)  InitialCondition=0  SampleTime=2.26757369614512e-05
  Rate Transition : hdlmdlgenlib/Buffer
      settings: SourceProductBaseCode=SL
  delayMatch : Delay  DelayLength=double(1)  InitialCondition=0  SampleTime=2.26757369614512e-05
  Out_HiD_o : Outport  OutDataTypeStr=fixdt(1,16,23)  SampleTime=2.26757369614512e-05  VectorParamsAs1DForOutWhenUnconnected=off
  wires:
  Add/1 -> Out_HiD_o/1
  Delay/1 -> Rate Transition/1
  HiD_1/1 -> HwModeRegister/1
  HiD_3/1 -> HwModeRegister2/1
  PipelineRegister/1 -> Add/1
  delayMatch/1 -> Add/2
  Rate Transition/1 -> HwModeRegister3/1
  In_HiD_o/1 -> Delay/1, HwModeRegister1/1
  PipelineRegister1/1 -> delayMatch/1
  Multiply/1 -> PipelineRegister/1
  HwModeRegister/1 -> Multiply/1
  HwModeRegister1/1 -> Multiply/2
  Multiply1/1 -> PipelineRegister1/1
  HwModeRegister2/1 -> Multiply1/1
  HwModeRegister3/1 -> Multiply1/2

== system gm_final_heart_sym2_level3_hdl/DWT_Sym2_Level3/1st_Level_Decomp/LoD_Even ==
  In_LoD_e : Inport  OutDataTypeStr=fixdt(0, 16, 23)  PortDimensions=1  SampleTime=2.26757369614512e-05
  Add : Sum  AccumDataTypeStr=fixdt(1, 16, 22)  OutDataTypeStr=fixdt(1, 16, 23)  SampleTime=2.26757369614512e-05
  Delay : Delay  DelayLength=double(1)  InitialCondition=0  SampleTime=2.26757369614512e-05
  HwModeRegister{,1..3} (4 alike) : Delay  DelayLength=double(1)  InitialCondition=0  SampleTime=2.26757369614512e-05
  LoD_0 : Constant  Value=-0.1294097900390625  OutDataTypeStr=fixdt(1, 16, 17)  SampleTime=2.26757369614512e-05
  LoD_2 : Constant  Value=0.836517333984375  OutDataTypeStr=fixdt(0, 16, 16)  SampleTime=2.26757369614512e-05
  Multiply : Product  Inputs=**  OutDataTypeStr=fixdt(1, 16, 15)  SampleTime=2.26757369614512e-05
  Multiply1 : Product  Inputs=**  OutDataTypeStr=fixdt(0, 16, 23)  SampleTime=2.26757369614512e-05
  PipelineRegister : Delay  DelayLength=double(1)  InitialCondition=0  SampleTime=2.26757369614512e-05
  PipelineRegister1 : Delay  DelayLength=double(1)  InitialCondition=0  SampleTime=2.26757369614512e-05
  Rate Transition : hdlmdlgenlib/Buffer
      settings: SourceProductBaseCode=SL
  delayMatch : Delay  DelayLength=double(1)  InitialCondition=0  SampleTime=2.26757369614512e-05
  Out_LoD_e : Outport  OutDataTypeStr=fixdt(1,16,23)  SampleTime=2.26757369614512e-05  VectorParamsAs1DForOutWhenUnconnected=off
  wires:
  Add/1 -> Out_LoD_e/1
  Delay/1 -> Rate Transition/1
  LoD_0/1 -> HwModeRegister/1
  LoD_2/1 -> HwModeRegister2/1
  PipelineRegister/1 -> Add/1
  delayMatch/1 -> Add/2
  Rate Transition/1 -> HwModeRegister3/1
  In_LoD_e/1 -> Delay/1, HwModeRegister1/1
  PipelineRegister1/1 -> delayMatch/1
  Multiply/1 -> PipelineRegister/1
  HwModeRegister/1 -> Multiply/1
  HwModeRegister1/1 -> Multiply/2
  Multiply1/1 -> PipelineRegister1/1
  HwModeRegister2/1 -> Multiply1/1
  HwModeRegister3/1 -> Multiply1/2

== system gm_final_heart_sym2_level3_hdl/DWT_Sym2_Level3/1st_Level_Decomp/LoD_Odd ==
  In_LoD_o : Inport  OutDataTypeStr=fixdt(0, 16, 23)  PortDimensions=1  SampleTime=2.26757369614512e-05
  Add : Sum  AccumDataTypeStr=fixdt(0, 16, 24)  OutDataTypeStr=fixdt(0, 16, 24)  SampleTime=2.26757369614512e-05
  Delay : Delay  DelayLength=double(1)  InitialCondition=0  SampleTime=2.26757369614512e-05
  HwModeRegister{,1..3} (4 alike) : Delay  DelayLength=double(1)  InitialCondition=0  SampleTime=2.26757369614512e-05
  LoD_1 : Constant  Value=0.22414398193359375  OutDataTypeStr=fixdt(0, 16, 18)  SampleTime=2.26757369614512e-05
  LoD_3 : Constant  Value=0.48296356201171875  OutDataTypeStr=fixdt(0, 16, 17)  SampleTime=2.26757369614512e-05
  Multiply : Product  Inputs=**  OutDataTypeStr=fixdt(0, 16, 25)  SampleTime=2.26757369614512e-05
  Multiply1 : Product  Inputs=**  OutDataTypeStr=fixdt(0, 16, 24)  SampleTime=2.26757369614512e-05
  PipelineRegister : Delay  DelayLength=double(1)  InitialCondition=0  SampleTime=2.26757369614512e-05
  PipelineRegister1 : Delay  DelayLength=double(1)  InitialCondition=0  SampleTime=2.26757369614512e-05
  Rate Transition : hdlmdlgenlib/Buffer
      settings: SourceProductBaseCode=SL
  delayMatch : Delay  DelayLength=double(1)  InitialCondition=0  SampleTime=2.26757369614512e-05
  Out_LoD_o : Outport  OutDataTypeStr=fixdt(0,16,24)  SampleTime=2.26757369614512e-05  VectorParamsAs1DForOutWhenUnconnected=off
  wires:
  Add/1 -> Out_LoD_o/1
  Delay/1 -> Rate Transition/1
  LoD_1/1 -> HwModeRegister/1
  LoD_3/1 -> HwModeRegister2/1
  PipelineRegister/1 -> Add/1
  delayMatch/1 -> Add/2
  Rate Transition/1 -> HwModeRegister3/1
  In_LoD_o/1 -> Delay/1, HwModeRegister1/1
  PipelineRegister1/1 -> delayMatch/1
  Multiply/1 -> PipelineRegister/1
  HwModeRegister/1 -> Multiply/1
  HwModeRegister1/1 -> Multiply/2
  Multiply1/1 -> PipelineRegister1/1
  HwModeRegister2/1 -> Multiply1/1
  HwModeRegister3/1 -> Multiply1/2

== system gm_final_heart_sym2_level3_hdl/DWT_Sym2_Level3/1st_Level_Decomp1/HiD_Even ==
  In_HiD_e : Inport  OutDataTypeStr=fixdt(1, 16, 22)  PortDimensions=1  SampleTime=2.26757369614512e-05
  Add : Sum  AccumDataTypeStr=fixdt(1, 16, 15)  OutDataTypeStr=fixdt(1, 16, 15)  SampleTime=2.26757369614512e-05
  Delay : Delay  DelayLength=double(1)  InitialCondition=0  SampleTime=2.26757369614512e-05
  HiD_0 : Constant  Value=-0.4829559326171875  OutDataTypeStr=fixdt(1, 16, 16)  SampleTime=2.26757369614512e-05
  HiD_2 : Constant  Value=-0.22414398193359375  OutDataTypeStr=fixdt(1, 16, 17)  SampleTime=2.26757369614512e-05
  HwModeRegister{,1..3} (4 alike) : Delay  DelayLength=double(1)  InitialCondition=0  SampleTime=2.26757369614512e-05
  Multiply : Product  Inputs=**  OutDataTypeStr=fixdt(1, 16, 15)  SampleTime=2.26757369614512e-05
  Multiply1 : Product  Inputs=**  OutDataTypeStr=fixdt(1, 16, 15)  SampleTime=2.26757369614512e-05
  PipelineRegister : Delay  DelayLength=double(1)  InitialCondition=0  SampleTime=2.26757369614512e-05
  PipelineRegister1 : Delay  DelayLength=double(1)  InitialCondition=0  SampleTime=2.26757369614512e-05
  Rate Transition : hdlmdlgenlib/Buffer
      settings: SourceProductBaseCode=SL
  delayMatch : Delay  DelayLength=double(1)  InitialCondition=0  SampleTime=2.26757369614512e-05
  Out_HiD_e : Outport  OutDataTypeStr=fixdt(1,16,15)  SampleTime=2.26757369614512e-05  VectorParamsAs1DForOutWhenUnconnected=off
  wires:
  Add/1 -> Out_HiD_e/1
  Delay/1 -> Rate Transition/1
  HiD_0/1 -> HwModeRegister/1
  HiD_2/1 -> HwModeRegister2/1
  PipelineRegister/1 -> Add/1
  delayMatch/1 -> Add/2
  Rate Transition/1 -> HwModeRegister3/1
  In_HiD_e/1 -> Delay/1, HwModeRegister1/1
  PipelineRegister1/1 -> delayMatch/1
  Multiply/1 -> PipelineRegister/1
  HwModeRegister/1 -> Multiply/1
  HwModeRegister1/1 -> Multiply/2
  Multiply1/1 -> PipelineRegister1/1
  HwModeRegister2/1 -> Multiply1/1
  HwModeRegister3/1 -> Multiply1/2

== system gm_final_heart_sym2_level3_hdl/DWT_Sym2_Level3/1st_Level_Decomp1/HiD_Odd ==
  In_HiD_o : Inport  OutDataTypeStr=fixdt(1, 16, 22)  PortDimensions=1  SampleTime=2.26757369614512e-05
  Add : Sum  AccumDataTypeStr=fixdt(1, 16, 23)  OutDataTypeStr=fixdt(1, 16, 23)  SampleTime=2.26757369614512e-05
  Delay : Delay  DelayLength=double(1)  InitialCondition=0  SampleTime=2.26757369614512e-05
  HiD_1 : Constant  Value=0.836517333984375  OutDataTypeStr=fixdt(0, 16, 16)  SampleTime=2.26757369614512e-05
  HiD_3 : Constant  Value=-0.1294097900390625  OutDataTypeStr=fixdt(1, 16, 17)  SampleTime=2.26757369614512e-05
  HwModeRegister{,1..3} (4 alike) : Delay  DelayLength=double(1)  InitialCondition=0  SampleTime=2.26757369614512e-05
  Multiply : Product  Inputs=**  OutDataTypeStr=fixdt(0, 16, 24)  SampleTime=2.26757369614512e-05
  Multiply1 : Product  Inputs=**  OutDataTypeStr=fixdt(1, 16, 15)  SampleTime=2.26757369614512e-05
  PipelineRegister : Delay  DelayLength=double(1)  InitialCondition=0  SampleTime=2.26757369614512e-05
  PipelineRegister1 : Delay  DelayLength=double(1)  InitialCondition=0  SampleTime=2.26757369614512e-05
  Rate Transition : hdlmdlgenlib/Buffer
      settings: SourceProductBaseCode=SL
  delayMatch : Delay  DelayLength=double(1)  InitialCondition=0  SampleTime=2.26757369614512e-05
  Out_HiD_o : Outport  OutDataTypeStr=fixdt(1,16,23)  SampleTime=2.26757369614512e-05  VectorParamsAs1DForOutWhenUnconnected=off
  wires:
  Add/1 -> Out_HiD_o/1
  Delay/1 -> Rate Transition/1
  HiD_1/1 -> HwModeRegister/1
  HiD_3/1 -> HwModeRegister2/1
  PipelineRegister/1 -> Add/1
  delayMatch/1 -> Add/2
  Rate Transition/1 -> HwModeRegister3/1
  In_HiD_o/1 -> Delay/1, HwModeRegister1/1
  PipelineRegister1/1 -> delayMatch/1
  Multiply/1 -> PipelineRegister/1
  HwModeRegister/1 -> Multiply/1
  HwModeRegister1/1 -> Multiply/2
  Multiply1/1 -> PipelineRegister1/1
  HwModeRegister2/1 -> Multiply1/1
  HwModeRegister3/1 -> Multiply1/2

== system gm_final_heart_sym2_level3_hdl/DWT_Sym2_Level3/1st_Level_Decomp1/LoD_Even ==
  In_LoD_e : Inport  OutDataTypeStr=fixdt(1, 16, 22)  PortDimensions=1  SampleTime=2.26757369614512e-05
  Add : Sum  AccumDataTypeStr=fixdt(1, 16, 23)  OutDataTypeStr=fixdt(1, 16, 23)  SampleTime=2.26757369614512e-05
  Delay : Delay  DelayLength=double(1)  InitialCondition=0  SampleTime=2.26757369614512e-05
  HwModeRegister{,1..3} (4 alike) : Delay  DelayLength=double(1)  InitialCondition=0  SampleTime=2.26757369614512e-05
  LoD_0 : Constant  Value=-0.1294097900390625  OutDataTypeStr=fixdt(1, 16, 17)  SampleTime=2.26757369614512e-05
  LoD_2 : Constant  Value=0.836517333984375  OutDataTypeStr=fixdt(0, 16, 16)  SampleTime=2.26757369614512e-05
  Multiply : Product  Inputs=**  OutDataTypeStr=fixdt(1, 16, 15)  SampleTime=2.26757369614512e-05
  Multiply1 : Product  Inputs=**  OutDataTypeStr=fixdt(0, 16, 24)  SampleTime=2.26757369614512e-05
  PipelineRegister : Delay  DelayLength=double(1)  InitialCondition=0  SampleTime=2.26757369614512e-05
  PipelineRegister1 : Delay  DelayLength=double(1)  InitialCondition=0  SampleTime=2.26757369614512e-05
  Rate Transition : hdlmdlgenlib/Buffer
      settings: SourceProductBaseCode=SL
  delayMatch : Delay  DelayLength=double(1)  InitialCondition=0  SampleTime=2.26757369614512e-05
  Out_LoD_e : Outport  OutDataTypeStr=fixdt(1,16,23)  SampleTime=2.26757369614512e-05  VectorParamsAs1DForOutWhenUnconnected=off
  wires:
  Add/1 -> Out_LoD_e/1
  Delay/1 -> Rate Transition/1
  LoD_0/1 -> HwModeRegister/1
  LoD_2/1 -> HwModeRegister2/1
  PipelineRegister/1 -> Add/1
  delayMatch/1 -> Add/2
  Rate Transition/1 -> HwModeRegister3/1
  In_LoD_e/1 -> Delay/1, HwModeRegister1/1
  PipelineRegister1/1 -> delayMatch/1
  Multiply/1 -> PipelineRegister/1
  HwModeRegister/1 -> Multiply/1
  HwModeRegister1/1 -> Multiply/2
  Multiply1/1 -> PipelineRegister1/1
  HwModeRegister2/1 -> Multiply1/1
  HwModeRegister3/1 -> Multiply1/2
